simulink model "LQR"  (R2020a)
settings: Solver=VariableStepAuto  StartTime=0.0  StopTime=10.0  RelTol=1e-3
settings Model: Creator=18423  LastModifiedBy=18423

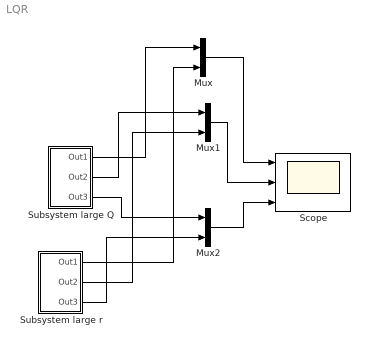
== system LQR ==
  Mux : Mux  Inputs=2
  Mux1 : Mux  Inputs=2
  Mux2 : Mux  Inputs=2
  Scope : Scope  NumInputPorts=3
  Subsystem large Q : Subsystem
  Subsystem large r : Subsystem
  wires:
  Subsystem large Q/1(Out1) -> Mux/1
  Subsystem large r/1(Out1) -> Mux/2
  Mux/1 -> Scope/1
  Subsystem large Q/2(Out2) -> Mux1/1
  Subsystem large r/2(Out2) -> Mux1/2
  Mux1/1 -> Scope/2
  Subsystem large Q/3(Out3) -> Mux2/1
  Subsystem large r/3(Out3) -> Mux2/2
  Mux2/1 -> Scope/3

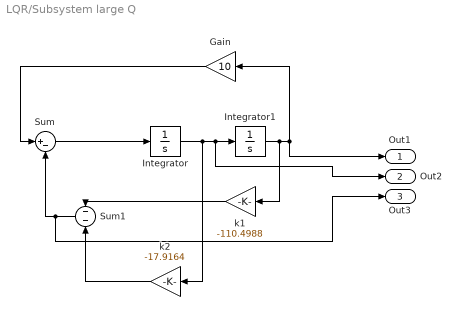
== system LQR/Subsystem large Q ==
  Gain : Gain  Gain=10
  Integrator : Integrator
  Integrator1 : Integrator  InitialCondition=5
  Sum : Sum  Inputs=|+-
  Sum1 : Sum  Inputs=--
  k1 : Gain  Gain=-110.4988
  k2 : Gain  Gain=-17.9164
  Out1 : Outport
  Out2 : Outport  Port=2
  Out3 : Outport  Port=3
  wires:
  Sum/1 -> Integrator/1
  Sum1/1 -> Out3/1, Sum/2
  Integrator1/1 -> k1/1, Out1/1, Gain/1
  Integrator/1 -> k2/1, Out2/1, Integrator1/1
  k2/1 -> Sum1/2
  Gain/1 -> Sum/1
  k1/1 -> Sum1/1

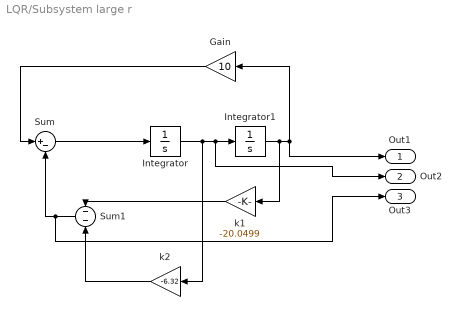
== system LQR/Subsystem large r ==
  Gain : Gain  Gain=10
  Integrator : Integrator
  Integrator1 : Integrator  InitialCondition=5
  Sum : Sum  Inputs=|+-
  Sum1 : Sum  Inputs=--
  k1 : Gain  Gain=-20.0499
  k2 : Gain  Gain=-6.32
  Out1 : Outport
  Out2 : Outport  Port=2
  Out3 : Outport  Port=3
  wires:
  Sum/1 -> Integrator/1
  Sum1/1 -> Out3/1, Sum/2
  Integrator1/1 -> k1/1, Out1/1, Gain/1
  Integrator/1 -> k2/1, Out2/1, Integrator1/1
  k2/1 -> Sum1/2
  Gain/1 -> Sum/1
  k1/1 -> Sum1/1
